simulink model "Posture_Regulation_Singularity"  (R2022b)
settings: Solver=FixedStepAuto  StartTime=0.0  StopTime=10.0  MaxStep=0.1  RelTol=1e-3
undefined symbols (not defined in the file): theta_f, unicycle, x_f, y_f
libraries: simulink_extras x2, dspsigops x1
settings Model: Creator=Musta  LastModifiedBy=Musta

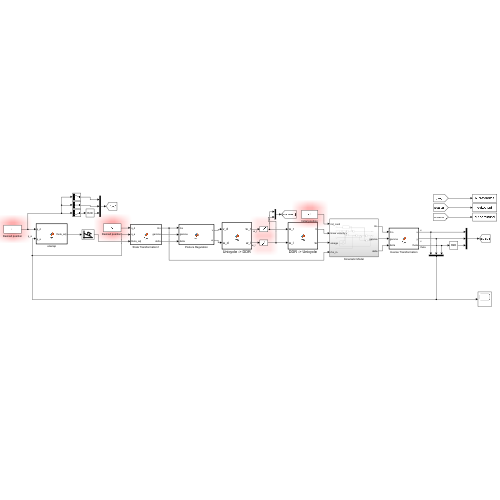
[thumbnail: Simulink's stored preview of the top-level diagram]
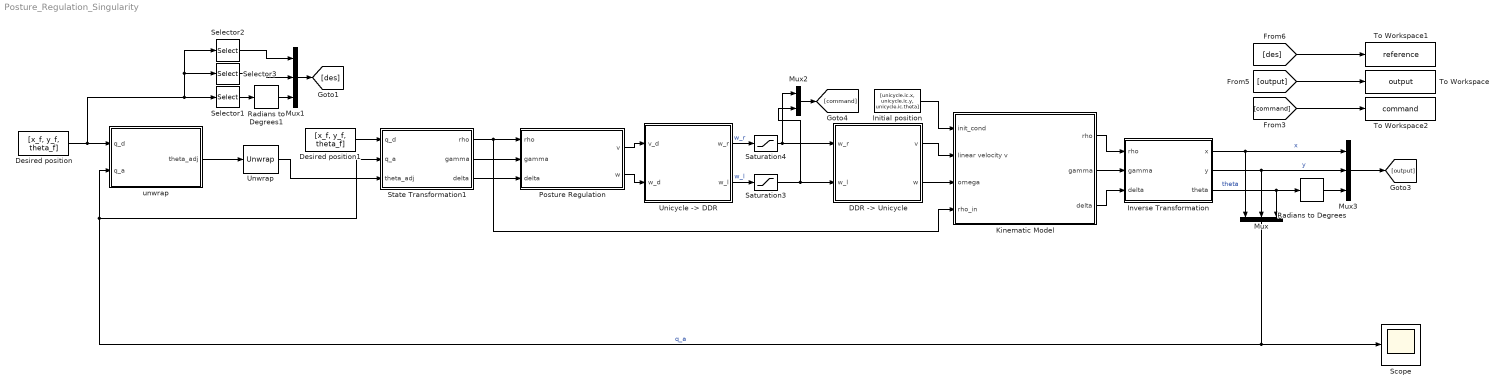
== system Posture_Regulation_Singularity ==
  " DDR -> Unicycle " : MATLAB Function  TreatAsAtomicUnit=on
  Desired position : Constant  Value=[x_f, y_f, theta_f]
  Desired position1 : Constant  Value=[x_f, y_f, theta_f]
  Initial position : Constant  Value=[unicycle.ic.x, unicycle.ic.y, unicycle.ic.theta]
  Inverse Transformation : MATLAB Function  TreatAsAtomicUnit=on
  Kinematic Model : Subsystem
  Mux : Mux  Inputs=3
  Mux1 : Mux  Inputs=3
  Mux2 : Mux  Inputs=2
  Mux3 : Mux  Inputs=3
  Posture Regulation : MATLAB Function  TreatAsAtomicUnit=on
  Radians to Degrees : simulink_extras/Transformations/Radians to Degrees
  Radians to Degrees1 : simulink_extras/Transformations/Radians to Degrees
  Saturation3 : Saturate  UpperLimit=unicycle.omegaWheelMax  LowerLimit=unicycle.omegaWheelMin
  Saturation4 : Saturate  UpperLimit=unicycle.omegaWheelMax  LowerLimit=unicycle.omegaWheelMin
  Scope : Scope
  Selector1 : Selector  InputPortWidth=3  IndexOptions=Index vector (dialog)  Indices=3  OutputSizes=1
  Selector2 : Selector  InputPortWidth=3  IndexOptions=Index vector (dialog)  Indices=1  OutputSizes=1
  Selector3 : Selector  InputPortWidth=3  IndexOptions=Index vector (dialog)  Indices=2  OutputSizes=1
  State Transformation1 : MATLAB Function  TreatAsAtomicUnit=on
  To Workspace : ToWorkspace  VariableName=output  SaveFormat=Structure With Time  SampleTime=-1
  To Workspace1 : ToWorkspace  VariableName=reference  SaveFormat=Structure With Time  SampleTime=-1
  To Workspace2 : ToWorkspace  VariableName=command  SaveFormat=Structure With Time  SampleTime=-1
  "Unicycle -> DDR" : MATLAB Function  TreatAsAtomicUnit=on
  Unwrap : dspsigops/Unwrap  tol=pi  InputProcessing=Columns as channels (frame based)  running=off
  unwrap : MATLAB Function  TreatAsAtomicUnit=on
  wires:
  Selector2/1 -> Mux1/1
  [output] -> To Workspace/1
  Selector1/1 -> Radians to Degrees1/1
  [command] -> To Workspace2/1
  Selector3/1 -> Mux1/2
  Posture Regulation/2(w) -> "Unicycle -> DDR"/2(w_d)
  Radians to Degrees1/1 -> Mux1/3
  [des] -> To Workspace1/1
  Desired position/1 -> Selector2/1, Selector3/1, Selector1/1, unwrap/1(q_d)
  Mux1/1 -> [des]
  Mux/1 -> State Transformation1/2(q_a), unwrap/2(q_a), Scope/1  "q_a"
  Posture Regulation/1(v) -> "Unicycle -> DDR"/1(v_d)
  Radians to Degrees/1 -> Mux3/3
  Mux3/1 -> [output]
  " DDR -> Unicycle "/1(v) -> Kinematic Model/2(linear velocity v)
  Mux2/1 -> [command]
  " DDR -> Unicycle "/2(w) -> Kinematic Model/3(omega)
  Inverse Transformation/1(x) -> Mux/1, Mux3/1  "x"
  Inverse Transformation/2(y) -> Mux3/2, Mux/2  "y"
  Inverse Transformation/3(theta) -> Mux/3, Radians to Degrees/1  "theta"
  Initial position/1 -> Kinematic Model/1(init_cond)
  Kinematic Model/3(delta) -> Inverse Transformation/3(delta)
  Kinematic Model/1(rho) -> Inverse Transformation/1(rho)
  Kinematic Model/2(gamma) -> Inverse Transformation/2(gamma)
  "Unicycle -> DDR"/2(w_l) -> Saturation3/1  "w_l"
  Saturation4/1 -> " DDR -> Unicycle "/1(w_r), Mux2/1
  Saturation3/1 -> Mux2/2, " DDR -> Unicycle "/2(w_l)
  "Unicycle -> DDR"/1(w_r) -> Saturation4/1  "w_r"
  State Transformation1/1(rho) -> Kinematic Model/4(rho_in), Posture Regulation/1(rho)
  State Transformation1/2(gamma) -> Posture Regulation/2(gamma)
  State Transformation1/3(delta) -> Posture Regulation/3(delta)
  unwrap/1(theta_adj) -> Unwrap/1
  Unwrap/1 -> State Transformation1/3(theta_adj)
  Desired position1/1 -> State Transformation1/1(q_d)

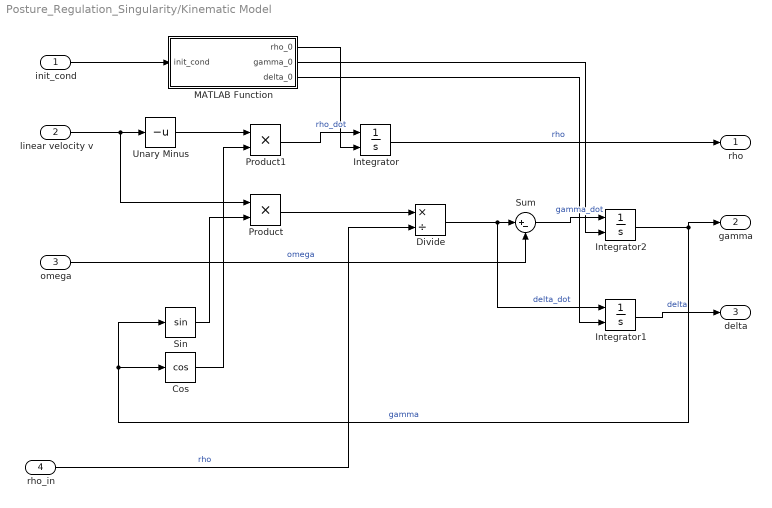
== system Posture_Regulation_Singularity/Kinematic Model ==
  init_cond : Inport
  linear velocity v : Inport  Port=2
  omega : Inport  Port=3
  rho_in : Inport  Port=4
  Cos : Trigonometry  Operator=cos
  Divide : Product  Inputs=*/
  Integrator : Integrator  InitialConditionSource=external
  Integrator1 : Integrator  InitialConditionSource=external
  Integrator2 : Integrator  InitialConditionSource=external
  MATLAB Function : MATLAB Function  TreatAsAtomicUnit=on
  Product : Product
  Product1 : Product
  Sin : Trigonometry
  Sum : Sum  Inputs=|+-
  Unary Minus : UnaryMinus
  rho : Outport
  gamma : Outport  Port=2
  delta : Outport  Port=3
  wires:
  Sum/1 -> Integrator2/1  "gamma_dot"
  Cos/1 -> Product1/2
  Unary Minus/1 -> Product1/1
  linear velocity v/1 -> Product/1, Unary Minus/1
  Product1/1 -> Integrator/1  "rho_dot"
  Integrator/1 -> rho/1  "rho"
  Sin/1 -> Product/2
  Product/1 -> Divide/1
  Divide/1 -> Integrator1/1, Sum/1  "delta_dot"
  omega/1 -> Sum/2  "omega"
  Integrator2/1 -> gamma/1, Cos/1, Sin/1  "gamma"
  Integrator1/1 -> delta/1  "delta"
  rho_in/1 -> Divide/2  "rho"
  init_cond/1 -> MATLAB Function/1(init_cond)
  MATLAB Function/1(rho_0) -> Integrator/2
  MATLAB Function/2(gamma_0) -> Integrator2/2
  MATLAB Function/3(delta_0) -> Integrator1/2

== matlab function Posture_Regulation_Singularity/State Transformation1 ==
  data: q_d input; rho output; q_a input; gamma output; delta output; theta_adj input
function [rho,gamma,delta] = fcn(q_d, q_a, theta_adj)

    e_x = q_d(1) - q_a(1);
    e_y = q_d(2) - q_a(2);
    e_theta = q_d(3) - q_a(3);
   
    rho = sqrt(e_x^2 + e_y^2);
    gamma = theta_adj - q_a(3);
    delta = gamma - e_theta;

end

== matlab function Posture_Regulation_Singularity/unwrap ==
  data: q_d input; theta_adj output; q_a input
function theta_adj = fcn(q_d, q_a)

    e_x = q_d(1) - q_a(1);
    e_y = q_d(2) - q_a(2);
    e_theta = q_d(3) - q_a(3);

    theta_adj = atan2(e_y,e_x);

end

== matlab function Posture_Regulation_Singularity/Posture Regulation ==
  data: v output; w output; rho input; gamma input; delta input
function [v,w] = fcn(rho,gamma,delta)

    %#codegen
    coder.extrinsic('evalin')
    k1 = 0;                  % Needed in order to set variable class correctly
    k2 = 0;                  % Needed in order to set variable class correctly
    k3 = 0;                  % Needed in order to set variable class correctly
    k1 = evalin('base','k1'); % Read value from workspace
    k2 = evalin('base','k2'); % Read value from workspace
    k3 = evalin('base','k3'); % Read value from workspace

    v = k1 * rho * cos(gamma);
    w = k2 * gamma + k1 *(sin(gamma)*cos(gamma))*(gamma + k3 * delta)/gamma;

    % handling the singularity of v 
    if abs(v) < 10^-4
        if v > 0
            v = 10^-4;
        else
            v = -10^-4;
        end   
    end    

end

== matlab function Posture_Regulation_Singularity/ DDR -> Unicycle  ==
  data: w_r input; v output; w_l input; w output
function [v, w] = fcn(w_r, w_l)

    %#codegen
    coder.extrinsic('evalin')
    d = 0;                  % Needed in order to set variable class correctly
    r = 0;                  % Needed in order to set variable class correctly
    d = evalin('base','unicycle.d'); % Read value from workspace
    r = evalin('base','unicycle.r'); % Read value from workspace

    v = r*(w_r + w_l)/2; % rad/s
    w = r*(w_r - w_l)/d; % rad/s

end

== matlab function Posture_Regulation_Singularity/Inverse Transformation ==
  data: x output; rho input; y output; gamma input; delta input; theta output
function [x,y,theta] = fcn(rho,gamma,delta)

    x = - rho * cos(delta);
    y = - rho * sin(delta);
    theta = delta - gamma;
    
end

== matlab function Posture_Regulation_Singularity/Kinematic Model/MATLAB Function ==
  data: init_cond input; rho_0 output; gamma_0 output; delta_0 output
function [rho_0, gamma_0, delta_0] = fcn(init_cond)

x_0 = init_cond(1);
y_0 = init_cond(2);
theta_0 = init_cond(3);


rho_0 = sqrt(x_0^2 + y_0^2);
gamma_0 = atan2(y_0,x_0) - theta_0 + pi;
delta_0 = gamma_0 + theta_0;

== matlab function Posture_Regulation_Singularity/Unicycle -> DDR ==
  data: v_d input; w_r output; w_d input; w_l output
function [w_r, w_l] = fcn(v_d, w_d)

    %#codegen
    coder.extrinsic('evalin')
    d = 0;                  % Needed in order to set variable class correctly
    r = 0;                  % Needed in order to set variable class correctly
    d = evalin('base','unicycle.d'); % Read value from workspace
    r = evalin('base','unicycle.r'); % Read value from workspace

    w_r = ((2 * v_d) + (w_d * d)) / (2 * r);
    w_l = ((2 * v_d) - (w_d * d)) / (2 * r);

end
